simulink model "nolinear_adaptive_controller"  (R2023a)
settings: Solver=VariableStepAuto  StartTime=0.0  StopTime=50  RelTol=1e-3
settings Model: Creator=belov  LastModifiedBy=belov

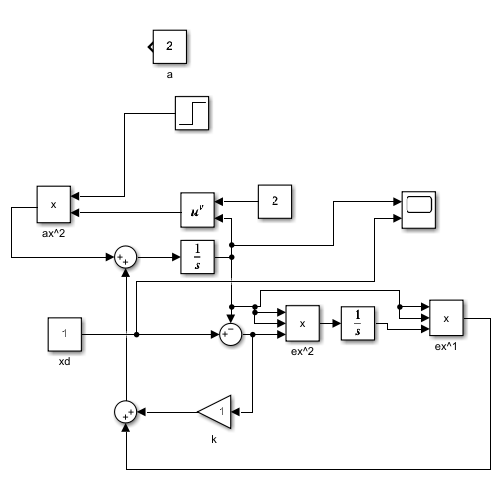
[thumbnail: Simulink's stored preview of the top-level diagram]
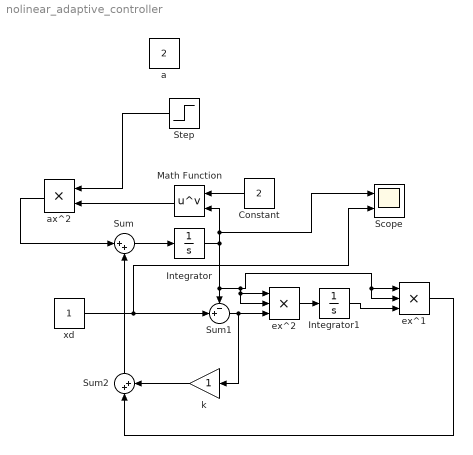
== system nolinear_adaptive_controller ==
  Constant : Constant  Value=2
  Integrator : Integrator
  Integrator1 : Integrator
  Math Function : Math  Operator=pow
  Scope : Scope  NumInputPorts=2
  Step : Step  Time=25  Before=1  After=2  SampleTime=0
  Sum : Sum  Inputs=|++
  Sum1 : Sum  Inputs=-+|
  Sum2 : Sum  Inputs=|++
  a : Constant  Value=2
  ax^2 : Product  Inputs=**
  ex^1 : Product  Inputs=***
  ex^2 : Product  Inputs=***
  k : Gain
  xd : Constant
  wires:
  Integrator/1 -> Scope/1, Math Function/2, Sum1/1, ex^1/2, ex^1/1, ex^2/2, ex^2/1
  Constant/1 -> Math Function/1
  Math Function/1 -> ax^2/2
  Sum/1 -> Integrator/1
  xd/1 -> Sum1/2, Scope/2
  Sum1/1 -> k/1, ex^2/3
  ex^2/1 -> Integrator1/1
  ax^2/1 -> Sum/1
  Integrator1/1 -> ex^1/3
  k/1 -> Sum2/2
  ex^1/1 -> Sum2/1
  Sum2/1 -> Sum/2
  Step/1 -> ax^2/1
